simulink model "Task8"  (R2022b)
settings: Solver=VariableStepAuto  StartTime=0.0  StopTime=10.0  RelTol=1e-3
settings Model: Creator=LOQ  LastModifiedBy=LOQ
settings OptimizationCC: ReuseModelBlockBuffer=on
settings RTWCC: GPUComputeCapability=5.0
settings ConfigComp: CovBoundaryAbsTol=1.0e-5

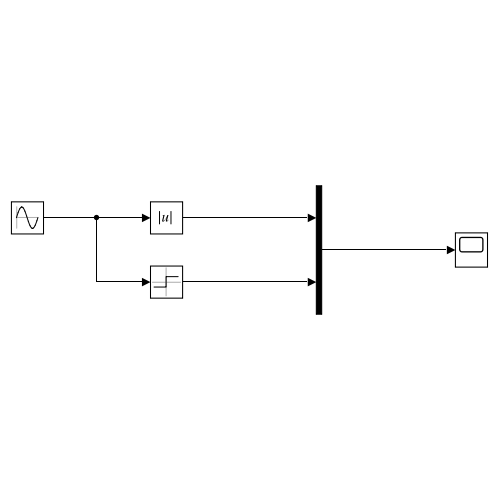
[thumbnail: Simulink's stored preview of the top-level diagram]
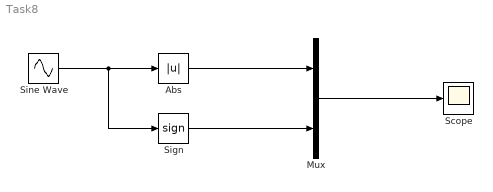
== system Task8 ==
  Abs : Abs  SaturateOnIntegerOverflow=off
  Mux : Mux  Inputs=2
  Scope : Scope
  Sign : Signum
  Sine Wave : Sin  SampleTime=0
  wires:
  Sine Wave/1 -> Sign/1, Abs/1
  Abs/1 -> Mux/1
  Sign/1 -> Mux/2
  Mux/1 -> Scope/1
